simulink model "verify_CondensingBoiler_mdl"  (R2016b)
settings: Solver=ode45  StartTime=0.0  StopTime=1800  MaxStep=10  RelTol=1e-3  EnableMultiTasking=on
libraries: carnot x5, simulink x1
settings Model: Creator=drhf  LastModifiedBy=drhf
settings DataIOCC: SaveFormat=Array
settings OptimizationCC: ExpressionDepthLimit=2147483647  LifeSpan=inf
settings DebuggingCC: UnderspecifiedInitializationDetection=Classic  MergeDetectMultiDrivingBlocksExec=none  SolverPrmCheckMsg=warning  StateNameClashWarn=warning  SFUnexpectedBacktrackingDiag=warning  SFNoUnconditionalDefaultTransitionDiag=warning  SFExecutionAtInitializationDiag=none
settings HardwareCC: ProdBitPerPointer=32  ProdBitPerSizeT=32  ProdBitPerPtrDiffT=32  ProdLargestAtomicFloat=None  ProdIntDivRoundTo=Undefined  ProdEndianess=Unspecified  ProdWordSize=32  ProdHWDeviceType=32-bit Generic
settings ModelReferenceCC: PropagateSignalLabelsOutOfModel=off
settings GRTTargetCC: TargetLangStandard=C89/C90 (ANSI)  GeneratePreprocessorConditionals=Disable all  CombineOutputUpdateFcns=off  GRTInterface=on
settings ConfigComp: CovMetricSettings=dw  CovHtmlReporting=on  CovSaveCumulativeToWorkspaceVar=on  CovSaveSingleToWorkspaceVar=on  CovExternalEMLEnable=off

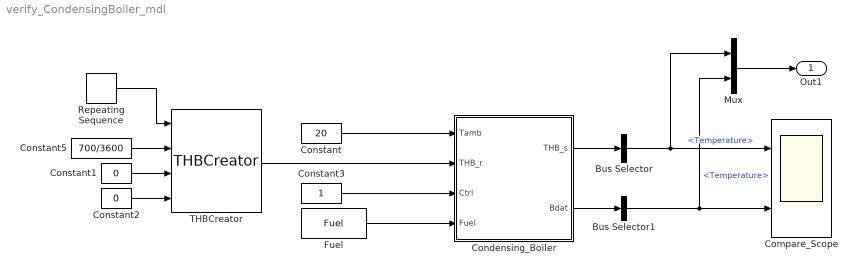
== system verify_CondensingBoiler_mdl ==
  Bus Selector : BusSelector  OutputSignals=Temperature
  Bus Selector1 : BusSelector  OutputSignals=THBin.Temperature
  Compare_Scope : Scope  NumInputPorts=2
  Condensing_Boiler : Subsystem  AncestorBlock=carnot/Source/Boiler/Condensing_Boiler  mask(Condensing Boiler){Pgas=15e3, U=3, vol=0.02, electricPower=[20 120], relativeQdot=[0.25 1], whichTforEfficiency=mean of inlet and outlet temperature, temperatures=[40  70], efficiency=[1.05 0.95; 1.0 0.9], lin=10, qua=100, Tini=20, nodes=1}
      mask prompts: Pgas "Heat input (= hi * GasMassflow) [W]"; U "heat loss coefficient [W/K]"; vol "volume of the boiler [m³]"; electricPower "Electric power in W (vector, index from relative power)"; relativeQdot "relative power in 0..1 (vector for row index)"; whichTforEfficiency "Efficiency table based on"; temperatures "Temperature in °C  (vector for column index)"; efficiency "Efficiency data in 0..1 (matrix)"; lin "pressure drop linear in massflow [Pa*s/kg]"; qua "pressure drop quadratic in massflow [Pa*s²/kg²]"; Tini "initial temperature [degree centigrade]"; nodes "number of nodes"
      mask help: Multinode one-dimensional model of a boiler. Condensing effects are taken in account by an efficiency lookup table.
      mask Help: web(fullfile(path_carnot('help'),'Condensing_Boiler.html'),'-helpbrowser')
      mask TypeOptions whichTforEfficiency: mean of inlet and outlet temperature | inlet temperature | outlet temperature
      mask Display: plot(-20,0,120,100,[10,90,90,10,10],[10,10,20,20,10],[80,80,20,20],[20,90,90,20],[20,70,70,20],[24,24,30,30],[32,30,28],[30,40,30],[43,40,38],[30,40,30],[53,50,47],[30,40,30],[63,60,57],[30,40,30],[35,32,30,29,31,36,39,40,37,35],[75,69,65,58,50,49,53,59,68,75],[57,54,51,51,53,58,62,62,59,57],[76,71,67,58,49,48,54,60,69,76])
  Constant : Constant  Value=20
  Constant1 : Constant  Value=0
  Constant2 : Constant  Value=0
  Constant3 : Constant
  Constant5 : Constant  Value=700/3600
  Fuel : carnot/Source/Energy/Fuel  ft=1  t=20  ls=3.5  p=1.013e5  h_values=[5.14e7 5.69e7]  tc=45  price=1  mass=[0.33 0.67 0 0 0 0]
  Mux : Mux  Inputs=2
  Repeating Sequence : simulink/Sources/Repeating Sequence  rep_seq_t="[0 200  1500 1801]"  rep_seq_y=[30 30 65 65]
  THBCreator : carnot/Basic/Hydraulics/THBCreator  Inport_ID=off  Inport_T=on  Inport_mdot=on  Inport_p=off  Inport_type=off  Inport_mix=off  Inport_mix2=on  Inport_mix3=on  Inport_d=off  Inport_c=off  Inport_l=off  Inport_q=off  Inport_LH=off  Inport_H=off  ID=20001  T=30  mdot=0  p=2e5  FluidType=1  FluidMix=0  FluidMix2=0  FluidMix3=0  d=0.02  c=0  l=0  q=0  LH=0  H=0  Annotation_ID=off  Annotation_T=off  Annotation_mdot=off  Annotation_p=off  Annotation_type=off  Annotation_mix=off  Annotation_mix2=off  Annotation_mix3=off  Annotation_d=off  Annotation_c=off  Annotation_l=off  Annotation_q=off  Annotation_LH=off  Annotation_H=off
  Out1 : Outport
  wires:
  Condensing_Boiler/1(THB_s) -> Bus Selector/1
  Bus Selector/1 -> Mux/1, Compare_Scope/1  "<Temperature>"
  Condensing_Boiler/2(Bdat) -> Bus Selector1/1
  Bus Selector1/1 -> Mux/2, Compare_Scope/2  "<Temperature>"
  Mux/1 -> Out1/1
  Constant5/1 -> THBCreator/2
  Repeating Sequence/1 -> THBCreator/1
  Constant/1 -> Condensing_Boiler/1(Tamb)
  THBCreator/1 -> Condensing_Boiler/2(THB_r)
  Fuel/1 -> Condensing_Boiler/4(Fuel)
  Constant3/1 -> Condensing_Boiler/3(Ctrl)
  Constant1/1 -> THBCreator/3
  Constant2/1 -> THBCreator/4

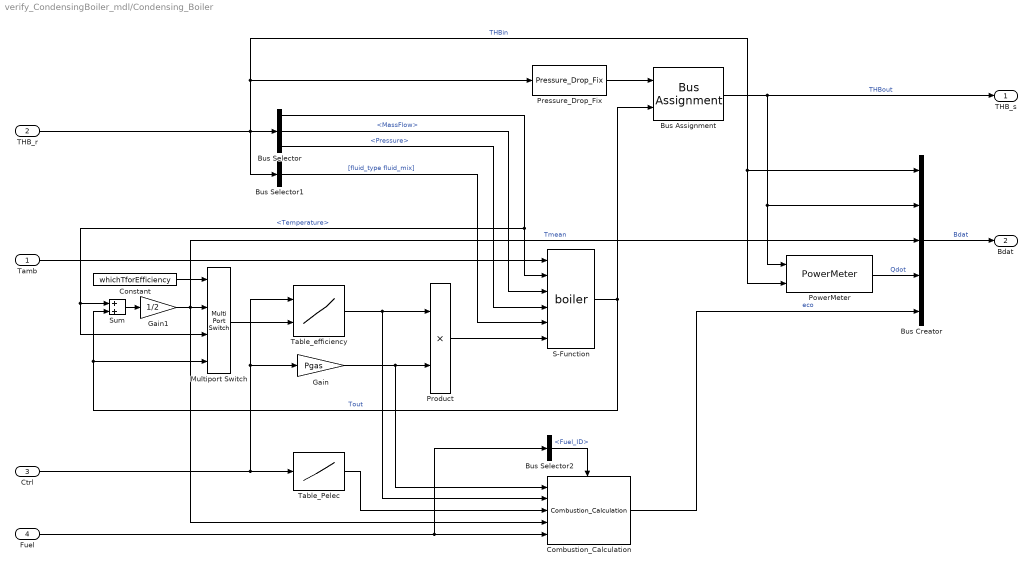
== system verify_CondensingBoiler_mdl/Condensing_Boiler ==
  Tamb : Inport
  THB_r : Inport  Port=2
  Ctrl : Inport  Port=3
  Fuel : Inport  Port=4
  Bus Assignment : BusAssignment  AssignedSignals=Temperature
  Bus Creator : BusCreator  Inputs=5
  Bus Selector : BusSelector  OutputSignals=Temperature,MassFlow,Pressure
  Bus Selector1 : BusSelector  OutputSignals=FluidType,FluidMix  OutputAsBus=on
  Bus Selector2 : BusSelector  OutputSignals=Fuel_ID
  Combustion_Calculation : carnot/Basic/Thermal_Models/Combustion_Calculation
  Constant : Constant  Value=whichTforEfficiency
  Gain : Gain  Gain=Pgas
  Gain1 : Gain  Gain=1/2
  Multiport Switch : MultiPortSwitch
  PowerMeter : carnot/Control/PowerMeter
  Pressure_Drop_Fix : carnot/Basic/Pressure_Drop/Pressure_Drop_Fix  con=0  lin=lin  qua=qua
  Product : Product  RndMeth=Zero
  S-Function : S-Function  FunctionName=boiler  Parameters=U,vol,Tini,nodes  SFunctionDeploymentMode=off  EnableBusSupport=off
  Sum : Sum
  Table_Pelec : Lookup_n-D  NumberOfTableDimensions=1  BreakpointsForDimension1=[0 relativeQdot]  Table=[0 electricPower]  InternalRulePriority=Speed  InputSameDT=on
  Table_efficiency : Lookup_n-D  BreakpointsForDimension1=relativeQdot  BreakpointsForDimension2=temperatures  Table=efficiency  InternalRulePriority=Speed
  THB_s : Outport
  Bdat : Outport  Port=2
  wires:
  Multiport Switch/1 -> Table_efficiency/2
  Constant/1 -> Multiport Switch/1
  Gain/1 -> Product/2, Combustion_Calculation/1
  Pressure_Drop_Fix/1 -> Bus Assignment/1
  Bus Selector2/1 -> Combustion_Calculation/Enable  "<Fuel_ID>"
  Product/1 -> S-Function/6
  Ctrl/1 -> Table_Pelec/1, Gain/1, Table_efficiency/1
  Table_efficiency/1 -> Product/1, Combustion_Calculation/2
  Fuel/1 -> Bus Selector2/1, Combustion_Calculation/5
  S-Function/1 -> Bus Assignment/2, Sum/2, Multiport Switch/4  "Tout"
  Bus Selector/1 -> S-Function/2, Sum/1, Multiport Switch/3  "<Temperature>"
  Tamb/1 -> S-Function/1
  Bus Selector/3 -> S-Function/4  "<Pressure>"
  Bus Assignment/1 -> PowerMeter/1, Bus Creator/2, THB_s/1  "THBout"
  Bus Selector/2 -> S-Function/3  "<MassFlow>"
  THB_r/1 -> PowerMeter/2, Bus Creator/1, Pressure_Drop_Fix/1, Bus Selector1/1, Bus Selector/1  "THBin"
  Bus Selector1/1 -> S-Function/5  "[fluid_type fluid_mix]"
  Bus Creator/1 -> Bdat/1  "Bdat"
  Gain1/1 -> Combustion_Calculation/4, Multiport Switch/2, Bus Creator/3  "Tmean"
  Table_Pelec/1 -> Combustion_Calculation/3
  PowerMeter/1 -> Bus Creator/4  "Qdot"
  Combustion_Calculation/1 -> Bus Creator/5  "eco"
  Sum/1 -> Gain1/1
